simulink model "Balancing_Robot_model"  (R2025a)
settings: Solver=ode23t  StartTime=0  StopTime=tspan(end)  MaxStep=1e-3  RelTol=1e-3  AbsTol=1e-3  EnableMultiTasking=on
InitFcn:
  | Balancing_Robot
values from neighbouring files (symbols this model uses):
  A_lin = double(subs(A_lin, 'upperLeg_theta', 0))    [Balancing_Robot.m]    (also in Inverted_pendulum_on_a_cart.m = double(A_lin); Inverted_pendulum_on_a_wheel.m = double(A_lin))
  B_lin = double(subs(B_lin, 'upperLeg_theta', 0))    [Balancing_Robot.m]    (also in Inverted_pendulum_on_a_cart.m = double(B_lin); Inverted_pendulum_on_a_wheel.m = double(B_lin))
  COM = struct    [Balancing_Robot.m]    (also in Copy_of_InvertedPendulum_Equations.m; InvertedPendulum_Equations_v1.m; Inverted_pendulum_on_a_cart.m; Inverted_pendulum_on_a_wheel.m)
  g = 9.80665    [Balancing_Robot.m]    (also in Copy_of_InvertedPendulum_Equations.m = 9.81; Gemini_trial_v2.m = 9.81; InvertedPendulum_Equations_v1.m = 9.81; Inverted_pendulum_on_a_cart.m = 9.81)
  K = lqr(A_lin, B_lin, Q, R)    [Balancing_Robot.m]    (also in Copy_of_InvertedPendulum_Equations.m = lqr(A, B, Q, R); Gemini_trial.m = lqr(A, B, Q, R); Gemini_trial_v2.m = lqr(A, B, Q, R); Inverted_pendulum_on_a_cart.m)
  lowerLeg = rod    [Balancing_Robot.m]    (also in Copy_of_InvertedPendulum_Equations.m = struct; InvertedPendulum_Equations_v1.m = struct; test_parameters.m = struct)
  m = 0.2    [Gemini_trial_v2.m]    (also in run_pendcart.m = 1)
  payload = struct    [Balancing_Robot.m]    (also in Copy_of_InvertedPendulum_Equations.m = 0)
  q0 = [0; 0]    [Balancing_Robot.m]    (also in Inverted_pendulum_on_a_cart.m; Inverted_pendulum_on_a_wheel.m)
  required_height = 0.8    [Balancing_Robot.m]
  rod = struct    [Balancing_Robot.m]    (also in Inverted_pendulum_on_a_cart.m; Inverted_pendulum_on_a_wheel.m)
  u_max = [tau_max; 0]    [Balancing_Robot.m]    (also in Inverted_pendulum_on_a_cart.m = [F_max; tau_max]; Inverted_pendulum_on_a_wheel.m)
  upperLeg = rod    [Balancing_Robot.m]    (also in Copy_of_InvertedPendulum_Equations.m = struct; InvertedPendulum_Equations_v1.m = struct; test_parameters.m = struct)
  wheel = struct    [Balancing_Robot.m]    (also in Copy_of_InvertedPendulum_Equations.m; InvertedPendulum_Equations_v1.m; Inverted_pendulum_on_a_wheel.m; test_parameters.m)
  wr = [6*pi; 0; 0; 0] + double([q0; q_dot0])    [Balancing_Robot.m]    (also in Copy_of_InvertedPendulum_Equations.m = [wheel.radius+floor.length/3; 0; 0; 0]; Inverted_pendulum_on_a_cart.m = [1; 0; 0; 0] + double([q0; q_dot0]); Inverted_pendulum_on_a_wheel.m; run_pendcart.m = [1; 0; pi; 0])
  x0 = x0 + double([q0; q_dot0])    [Balancing_Robot.m]    (also in Copy_of_InvertedPendulum_Equations.m = [0; 0; pi/2; pi/18]; InvertedPendulum_Equations_v1.m = [0; wheel.radius+lowerLeg.length-joint_offset; pi; 0]; Inverted_pendulum_on_a_cart.m = [-1; 0.5; 0; 0] + double([q0; q_dot0]); Inverted_pendulum_on_a_wheel.m = [0; -0.1; 0; 0] + double([q0; q_dot0]))
undefined symbols (not defined in the file or in its folder): C_pid, subs, X, Y, Z
libraries: sm_lib x50, nesl_utility x40, dspsigops x3, fl_lib x2, Wheel_Joint_Library x2, simulink x2, slpidlib x1
(part 3 of 3)

== matlab function Balancing_Robot_model/Reference Goal/MATLAB Function ==
  data: y_ref input; theta_ref output
function theta_ref = fcn(y_ref)
    % Initialization
    % We need two initial guesses to start the Secant method
    t0 = 0.1; 
    t1 = 0.2; 
    
    tol = 1e-5;      % How close to the answer is 'good enough'
    max_iter = 25;   % Safety break so the simulation doesn't freeze
    
    for i = 1:max_iter
        % CALL your Simulink Function here
        % Syntax: [out1, out2] = mySimulinkFunction(in1)
        y0 = height_function(t0); 
        y1 = height_function(t1);
        
        % Calculate the error (how far we are from y_ref)
        f0 = y0 - y_ref;
        f1 = y1 - y_ref;
        
        % Check if we are close enough
        if abs(f1) < tol
            break;
        end
        
        % Secant Method Formula: find the next guess
        % To avoid division by zero if f1 == f0
        if abs(f1 - f0) < 1e-12
            break;
        end
        
        t_next = t1 - f1 * (t1 - t0) / (f1 - f0);
        
        % Update guesses for the next loop
        t0 = t1;
        t1 = t_next;
    end
    
    theta_ref = t1;
end

== matlab function Balancing_Robot_model/LQR Control/MATLAB Function ==
  data: u_control input; u_saturated output; tau_max parameter
function u_saturated = fcn(u_control, tau_max)
u_saturated = max(-tau_max, min(tau_max, u_control));

== matlab function Balancing_Robot_model/Balancing Robot/Free Joint/calculate_COM_x ==
  data: wheel_theta input; out1 output; upperLeg_theta input; lowerLeg_theta input
function out1 = calculate_COM_x(wheel_theta,upperLeg_theta,lowerLeg_theta)
%#codegen

%    This function was generated by the Symbolic Math Toolbox version 25.1.
%    01-Jun-2026 02:56:31

% wheel_theta = complex(wheel_theta);  % if required to enforce complex operations
% upperLeg_theta = complex(upperLeg_theta);  % if required to enforce complex operations
% lowerLeg_theta = complex(lowerLeg_theta);  % if required to enforce complex operations
out1 = wheel_theta./1.0e+1+cos(lowerLeg_theta+upperLeg_theta).*2.895454545454545e-1+cos(lowerLeg_theta+pi./2.0).*1.813636363636364e-1;
end

== matlab function Balancing_Robot_model/Balancing Robot/Display COM/calculate_COM_x ==
  data: wheel_theta input; upperLeg_theta input; out1 output; lowerLeg_theta input
function out1 = calculate_COM_x(wheel_theta,upperLeg_theta,lowerLeg_theta)
%#codegen

%    This function was generated by the Symbolic Math Toolbox version 25.1.
%    29-May-2026 08:39:19

% wheel_theta = complex(wheel_theta);  % if required to enforce complex operations
% upperLeg_theta = complex(upperLeg_theta);  % if required to enforce complex operations
% lowerLeg_theta = complex(lowerLeg_theta);  % if required to enforce complex operations
out1 = wheel_theta./1.0e+1+cos(lowerLeg_theta+upperLeg_theta).*2.895454545454545e-1+cos(lowerLeg_theta+pi./2.0).*1.813636363636364e-1;
end

== matlab function Balancing_Robot_model/Sensor/calculate_COM_theta ==
  data: out1 output; upperLeg_theta input
function out1 = calculate_COM_theta(upperLeg_theta)
%#codegen

%    This function was generated by the Symbolic Math Toolbox version 25.1.
%    01-Jun-2026 02:56:31

% upperLeg_theta = complex(upperLeg_theta);  % if required to enforce complex operations
out1 = pi.*(-1.0./2.0)+atan2(sin(upperLeg_theta).*2.895454545454545e-1+1.813636363636364e-1,cos(upperLeg_theta).*2.895454545454545e-1);
end

== matlab function Balancing_Robot_model/Balancing Robot/Display COM/calculate_COM_y ==
  data: wheel_theta input; upperLeg_theta input; out1 output; lowerLeg_theta input
function out1 = calculate_COM_y(wheel_theta,upperLeg_theta,lowerLeg_theta)
%#codegen

%    This function was generated by the Symbolic Math Toolbox version 25.1.
%    29-May-2026 08:39:19

% wheel_theta = complex(wheel_theta);  % if required to enforce complex operations
% upperLeg_theta = complex(upperLeg_theta);  % if required to enforce complex operations
% lowerLeg_theta = complex(lowerLeg_theta);  % if required to enforce complex operations
out1 = sin(lowerLeg_theta+upperLeg_theta).*2.895454545454545e-1+sin(lowerLeg_theta+pi./2.0).*1.813636363636364e-1+1.0./1.0e+1;
end

== matlab function Balancing_Robot_model/Balancing Robot/Free Joint/calculate_COM_y ==
  data: wheel_theta input; out1 output; upperLeg_theta input; lowerLeg_theta input
function out1 = calculate_COM_y(wheel_theta,upperLeg_theta,lowerLeg_theta)
%#codegen

%    This function was generated by the Symbolic Math Toolbox version 25.1.
%    01-Jun-2026 02:56:31

% wheel_theta = complex(wheel_theta);  % if required to enforce complex operations
% upperLeg_theta = complex(upperLeg_theta);  % if required to enforce complex operations
% lowerLeg_theta = complex(lowerLeg_theta);  % if required to enforce complex operations
out1 = sin(lowerLeg_theta+upperLeg_theta).*2.895454545454545e-1+sin(lowerLeg_theta+pi./2.0).*1.813636363636364e-1+1.0./1.0e+1;
end
